simulink model "mech_pole_vault"  (Simulink 7.1)
settings: Solver=ode15s  StartTime=0.0  StopTime=5  RelTol=1e-3  AbsTol=1e-6
PreLoadFcn:
  | poleLength = 4; %m
  | poleAngle = 60;  %deg
  | poleMass = 12; %Kg
  | poleInertia = [11.9 0 0;0 11.9 0;0 0 0.0024];
  | %-----------------------------------------
  | jumperMass = 60; %Kg
  | jumperInertia = eye(3,3);
  | jumperCG = [0 -0.1 0];
  | %----------------------------------------
  | runLength = 10; %m
  | jumpHeight = 4; %m
InitFcn:
  | poleLength = 4; %m
  | poleAngle = 60;  %deg
  | poleMass = 12; %Kg
  | poleInertia = [11.9 0 0;0 11.9 0;0 0 0.0024];
  | %-----------------------------------------
  | jumperMass = 60; %Kg
  | jumperInertia = eye(3,3);
  | jumperCG = [0 -0.1 0];
  | %----------------------------------------
  | runLength = 10; %m
  | jumpHeight = 4; %m
undefined symbols (not defined in the file or in its folder): rad, s
libraries: mblibv1 x33, simulink x9
settings Model: Creator=arnav  LastModifiedBy=batserve
settings DataIOCC: OutputOption=SpecifiedOutputTimes  OutputTimes=linspace(0,5,100)  Refine=3
settings DebuggingCC: AlgebraicLoopMsg=none  SaveWithParameterizedLinksMsg=none  SignalResolutionControl=TryResolveAllWithWarning  SolverPrmCheckMsg=none  MultiTaskDSMMsg=warning  MultiTaskCondExecSysMsg=none  SigSpecEnsureSampleTimeMsg=none  ModelReferenceExtraNoncontSigs=warning  StrictBusMsg=None
settings HardwareCC: TargetBitPerLong=64  TargetEndianess=LittleEndian  TargetWordSize=64  TargetHWDeviceType=MATLAB Host  ProdEqTarget=off
settings RTWCC: SystemTargetFile=rsim.tlc  TemplateMakefile=rsim_default_tmf  Description=Rapid Simulation Target  ProcessScript=rsim_make_rtw_hook  IncludeERTFirstTime=on
settings RSimTargetCC: TargetFcnLib=ansi_tfl_tmw.mat  TargetFunctionLibrary=ANSI_C  IsPILTarget=off  EnableShiftOperators=on  PortableWordSizes=off
settings SimMechanicsCC: WarnOnRedundantConstraints=off  VisOnUpdateDiagram=on  VisDuringSimulation=on  VisConfigFile=mech_polevault.mat

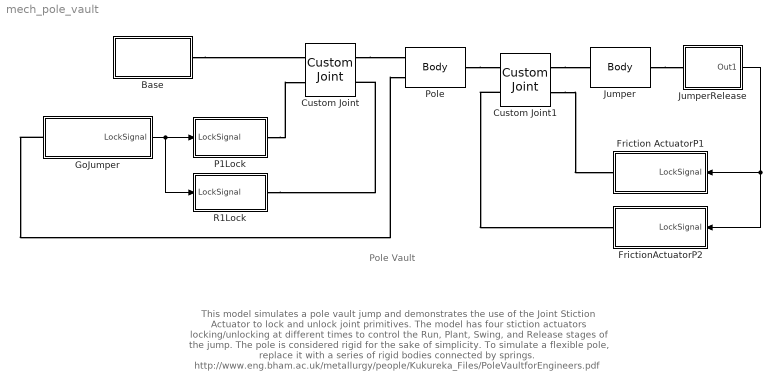
== system mech_pole_vault ==
  note: This model simulates a pole vault jump and demonstrates the use of
      | the Joint Stiction Actuator to lock and unlock joint primitives.
      | The model has four stiction actuators locking/unlocking at different times
      | to control the Run, Plant, Swing, and Release stages of the jump.
      |
      | The pole is considered rigid for the sake of simplicity.  To simulate a flexible pole,
      | replace it with a series of rigid bodies connected by springs.
      |
      | http://www.eng.bham.ac.uk/metallurgy/people/Kukureka_Files/PoleVaultforEngineers.pdf
  note: Pole Vault
  Base : Subsystem
  Custom Joint : mblibv1/Joints/Custom Joint  DialogController=MECH.DynMechDlgSource  PhysicalDomain=mechanical  SubClassName=custom_joint  LeftPortType=blob  RightPortType=blob  LConnTagsString=__newl0|SA1  RConnTagsString=__newr0|SA1  NumSAPorts=2  CutJoint=off  MarkAsCut=off  Primitives=prismatic_revolute  PrimitiveProps=P1$WORLD$[1 0 0]$prismatic#R1$WORLD$[0 0 1]$revolute  DialogClass=JointBlock  R1Axis=[0 0 1]  R2Axis=[]  R3Axis=[]  P1Axis=[1 0 0]  P2Axis=[]  P3Axis=[]  SAxis=[]
  Custom Joint1 : mblibv1/Joints/Custom Joint  DialogController=MECH.DynMechDlgSource  PhysicalDomain=mechanical  SubClassName=custom_joint  LeftPortType=blob  RightPortType=blob  LConnTagsString=__newl0|SA1  RConnTagsString=__newr0|SA1  NumSAPorts=2  CutJoint=off  MarkAsCut=off  Primitives=revolute_prismatic_prismatic  PrimitiveProps=R1$WORLD$[0 0 1]$revolute#P1$WORLD$[1 0 0]$prismatic#P2$WORLD$[0 1 0]$prismatic  DialogClass=JointBlock  R1Axis=[0 0 1]  R2Axis=[]  R3Axis=[]  P1Axis=[1 0 0]  P2Axis=[0 1 0]  P3Axis=[]  SAxis=[]
  Friction ActuatorP1 : Subsystem  Orientation=left  AncestorBlock=mech_friction/Normal Friction Actuator  mask(Normal Friction Actuator){Ckinetic=20, staticFF=20, Csforward=0.055, Csreverse=0.055, sExtActuation=on, sForces=off, primitive=P1}
      mask prompts: Ckinetic "Kinetic friction coefficient"; staticFF "Static friction coefficient"; Csforward "Forward stiction coefficient"; Csreverse "Reverse stiction coefficient"; sExtActuation "Show external actuation port"; sForces "Show kinetic and static friction ports"; primitive "Joint primitive"
      mask help:
      | Applies kinetic and static contact friction to a joint primitive. The friction force/torque is proportional to the force normal to the frictional surfaces in contact. In order for the actuated joint to be able to lock, the static friction coefficient muS must be larger than the kinetic friction coefficient muK. The friction force is mu*(normal force). The coefficient mu should be positive.
      |
      | Connect the round mechanical connection port to an actuator port on the Joint. You can friction actuate a prismatic or revolute primitive, but not a spherical primitive.
      |
      | The joint primitive menu lists all possible primitives. You must select the correct primitive after you connect the actuator to the joint.
      mask init:
      | Csforward = staticFF*Ckinetic;
      | Csreverse = staticFF*Ckinetic;
      | mech_normalFrictionActuator(gcb,'setPrimitive');
      | mech_normalFrictionActuator(gcb,'showHideActuatorSignal',sExtActuation);
      | mech_normalFrictionActuator(gcb,'showHideFrictionForces',sForces);
      settings: CopyFcn=|
      | %set_param(gcb,'LinkStatus','none');
      | %set_param(gcb,'CopyFcn','');
      mask StyleString: edit,edit,edit,edit,checkbox,checkbox,popup(P1|P2|P3|R1|R2|R3)
      mask CallbackString: ||||||%populateStictionPrimitiveList(gcb);
  FrictionActuatorP2 : Subsystem  Orientation=left  AncestorBlock=mech_friction/Normal Friction Actuator  mask(Normal Friction Actuator){Ckinetic=20, staticFF=20, Csforward=0.055, Csreverse=0.055, sExtActuation=on, sForces=off, primitive=P2}
      mask prompts: Ckinetic "Kinetic friction coefficient"; staticFF "Static friction coefficient"; Csforward "Forward stiction coefficient"; Csreverse "Reverse stiction coefficient"; sExtActuation "Show external actuation port"; sForces "Show kinetic and static friction ports"; primitive "Joint primitive"
      mask help:
      | Applies kinetic and static contact friction to a joint primitive. The friction force/torque is proportional to the force normal to the frictional surfaces in contact. In order for the actuated joint to be able to lock, the static friction coefficient muS must be larger than the kinetic friction coefficient muK. The friction force is mu*(normal force). The coefficient mu should be positive.
      |
      | Connect the round mechanical connection port to an actuator port on the Joint. You can friction actuate a prismatic or revolute primitive, but not a spherical primitive.
      |
      | The joint primitive menu lists all possible primitives. You must select the correct primitive after you connect the actuator to the joint.
      mask init: same as mech_pole_vault/Friction ActuatorP1
      settings: CopyFcn=|
      | %set_param(gcb,'LinkStatus','none');
      | %set_param(gcb,'CopyFcn','');
      mask StyleString: edit,edit,edit,edit,checkbox,checkbox,popup(P1|P2|P3|R1|R2|R3)
      mask CallbackString: ||||||%populateStictionPrimitiveList(gcb);
  GoJumper : Subsystem
  Jumper : mblibv1/Bodies/Body  DialogController=MECH.DynMechDlgSource  PhysicalDomain=mechanical  SubClassName=Unknown  LeftPortType=workingframe  RightPortType=workingframe  LConnTagsString=CS1  RConnTagsString=CG  DialogClass=MechanicalBodyBlock  Mass=jumperMass  MassUnits=kg  InertiaUnits=kg*m^2  Inertia=jumperInertia*1  Shape=Cylinder  ShapeDims=[1 1]  ShapeUnits=m  ShapeUse=false  Density=1  DensityUnits=kg/m^3  DensityUse=false  GraphicsMode=1  BodyColor=[0.5 0.5 0.5]  GraphicsObj=[]  AttachedToCS=1  CG=Right$CG$[0 -0.1 0]$CS1$CS1$m$[0 0 0]$Euler X-Y-Z$deg$WORLD$true  WorkingFrames=Left$CS1$[0 0 0]$ADJOINING$ADJOINING$m$[0 0 0]$Euler X-Y-Z$deg$WORLD$true#Right$CS2$[0 0 0]$CS1$CS1$m$[0 0 0]$Euler X-Y-Z$deg$WORLD$false  CGPos=[0 -0.1 0]  CGRot=[0 0 0]  CS0Pos=[]  CS0Rot=[]  CS1Pos=[0 0 0]  CS1Rot=[0 0 0]  CS2Pos=[0 0 0]  CS2Rot=[0 0 0]  CS3Pos=[]  CS3Rot=[]  CS4Pos=[]  CS4Rot=[]  CS5Pos=[]  CS5Rot=[]  CS6Pos=[]  CS6Rot=[]  CS7Pos=[]  CS7Rot=[]  CS8Pos=[]  CS8Rot=[]  CS9Pos=[]  CS9Rot=[]  CS10Pos=[]  CS10Rot=[]  CS11Pos=[]  CS11Rot=[]  CS12Pos=[]  CS12Rot=[]  CS13Pos=[]  CS13Rot=[]  CS14Pos=[]  CS14Rot=[]  CS15Pos=[]  CS15Rot=[]  CS16Pos=[]  CS16Rot=[]  CS17Pos=[]  CS17Rot=[]  CS18Pos=[]  CS18Rot=[]  CS19Pos=[]  CS19Rot=[]  CS20Pos=[]  CS20Rot=[]
  JumperRelease : Subsystem
  P1Lock : Subsystem
  Pole : mblibv1/Bodies/Body  DialogController=MECH.DynMechDlgSource  PhysicalDomain=mechanical  SubClassName=Unknown  LeftPortType=workingframe  RightPortType=workingframe  LConnTagsString=CS1|CS3  RConnTagsString=CS2  DialogClass=MechanicalBodyBlock  Mass=poleMass  MassUnits=kg  InertiaUnits=kg*m^2  Inertia=poleInertia  Shape=Cylinder  ShapeDims=[1 1]  ShapeUnits=m  ShapeUse=false  Density=1  DensityUnits=kg/m^3  DensityUse=false  GraphicsMode=1  BodyColor=[0.5 0.5 0.5]  GraphicsObj=[]  AttachedToCS=1  CG=Left$CG$[poleLength 0 0]/2$CS1$CS1$m$[0 90 0]$Euler X-Y-Z$deg$CS1$false  WorkingFrames=Left$CS1$[runLength 0 0]$WORLD$WORLD$m$[0 0 poleAngle]$Euler X-Y-Z$deg$WORLD$true#Left$CS3$[0 0 0]$CS1$CS1$m$[0 0 0]$Euler X-Y-Z$deg$WORLD$true#Right$CS2$[poleLength 0 0]$CS1$CS1$m$[0 0 0]$Euler X-Y-Z$deg$CS1$true  CGPos=[poleLength 0 0]/2  CGRot=[0 90 0]  CS0Pos=[]  CS0Rot=[]  CS1Pos=[runLength 0 0]  CS1Rot=[0 0 poleAngle]  CS2Pos=[poleLength 0 0]  CS2Rot=[0 0 0]  CS3Pos=[0 0 0]  CS3Rot=[0 0 0]  CS4Pos=[]  CS4Rot=[]  CS5Pos=[]  CS5Rot=[]  CS6Pos=[]  CS6Rot=[]  CS7Pos=[]  CS7Rot=[]  CS8Pos=[]  CS8Rot=[]  CS9Pos=[]  CS9Rot=[]  CS10Pos=[]  CS10Rot=[]  CS11Pos=[]  CS11Rot=[]  CS12Pos=[]  CS12Rot=[]  CS13Pos=[]  CS13Rot=[]  CS14Pos=[]  CS14Rot=[]  CS15Pos=[]  CS15Rot=[]  CS16Pos=[]  CS16Rot=[]  CS17Pos=[]  CS17Rot=[]  CS18Pos=[]  CS18Rot=[]  CS19Pos=[]  CS19Rot=[]  CS20Pos=[]  CS20Rot=[]
  R1Lock : Subsystem
  wires:
  GoJumper/1(LockSignal) -> R1Lock/1(LockSignal), P1Lock/1(LockSignal)
  JumperRelease/1(Out1) -> Friction ActuatorP1/1(LockSignal), FrictionActuatorP2/1(LockSignal)
  connections:
  Base/RConn1 -- Custom Joint/LConn1
  Custom Joint/RConn1 -- Pole/LConn1
  GoJumper/LConn1 -- Pole/LConn2
  Pole/RConn1 -- Custom Joint1/LConn1
  Custom Joint1/RConn1 -- Jumper/LConn1
  P1Lock/RConn1 -- Custom Joint/LConn2
  Jumper/RConn1 -- JumperRelease/LConn1
  R1Lock/RConn1 -- Custom Joint/RConn2
  Custom Joint1/RConn2 -- Friction ActuatorP1/RConn1
  Custom Joint1/LConn2 -- FrictionActuatorP2/RConn1

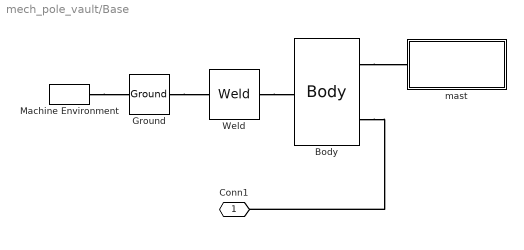
== system mech_pole_vault/Base ==
  Body : mblibv1/Bodies/Body  DialogController=MECH.DynMechDlgSource  PhysicalDomain=mechanical  SubClassName=Unknown  LeftPortType=workingframe  RightPortType=workingframe  LConnTagsString=CS1  RConnTagsString=CS4|CS2  DialogClass=MechanicalBodyBlock  Mass=30  MassUnits=kg  InertiaUnits=kg*m^2  Inertia=[1 0 0;0 0.01 0;0 0 1]*150  Shape=Cylinder  ShapeDims=[1 1]  ShapeUnits=m  ShapeUse=false  Density=1  DensityUnits=kg/m^3  DensityUse=false  GraphicsMode=1  BodyColor=[0.5 0.5 0.5]  GraphicsObj=[]  AttachedToCS=1  CG=Right$CG$[1 0 0]$CS1$CS1$m$[0 0 90]$Euler X-Y-Z$deg$WORLD$false  WorkingFrames=Right$CS4$[0 0 0]$CS1$CS1$m$[0 0 0]$Euler X-Y-Z$deg$WORLD$true#Left$CS1$[0 0 0]$ADJOINING$ADJOINING$m$[0 0 0]$Euler X-Y-Z$deg$WORLD$true#Right$CS2$[0 0 0]$CS1$CS1$m$[0 0 0]$Euler X-Y-Z$deg$WORLD$true#Right$CS3$[-3 0 0]$CS1$CS1$m$[0 0 0]$Euler X-Y-Z$deg$WORLD$false#Right$CS5$[-10 0 0]$CS1$CS1$m$[0 0 0]$Euler X-Y-Z$deg$WORLD$false#Right$CS6$[9 0 2]$CS1$CS1$m$[0 0 0]$Euler X-Y-Z$deg$WORLD$false#Right$CS7$[9 0 -2]$CS1$CS1$m$[0 0 0]$Euler X-Y-Z$deg$WORLD$false#Right$CS8$[-10 0 2]$CS1$CS1$m$[0 0 0]$Euler X-Y-Z$deg$WORLD$false#Right$CS9$[-10 0 -2]$CS1$CS1$m$[0 0 0]$Euler X-Y-Z$deg$WORLD$false  CGPos=[1 0 0]  CGRot=[0 0 90]  CS0Pos=[]  CS0Rot=[]  CS1Pos=[0 0 0]  CS1Rot=[0 0 0]  CS2Pos=[0 0 0]  CS2Rot=[0 0 0]  CS3Pos=[-3 0 0]  CS3Rot=[0 0 0]  CS4Pos=[0 0 0]  CS4Rot=[0 0 0]  CS5Pos=[-10 0 0]  CS5Rot=[0 0 0]  CS6Pos=[9 0 2]  CS6Rot=[0 0 0]  CS7Pos=[9 0 -2]  CS7Rot=[0 0 0]  CS8Pos=[-10 0 2]  CS8Rot=[0 0 0]  CS9Pos=[-10 0 -2]  CS9Rot=[0 0 0]  CS10Pos=[]  CS10Rot=[]  CS11Pos=[]  CS11Rot=[]  CS12Pos=[]  CS12Rot=[]  CS13Pos=[]  CS13Rot=[]  CS14Pos=[]  CS14Rot=[]  CS15Pos=[]  CS15Rot=[]  CS16Pos=[]  CS16Rot=[]  CS17Pos=[]  CS17Rot=[]  CS18Pos=[]  CS18Rot=[]  CS19Pos=[]  CS19Rot=[]  CS20Pos=[]  CS20Rot=[]
  Ground : mblibv1/Bodies/Ground  DialogController=MECH.DynMechDlgSource  SystemSampleTime=-1  LeftPortType=env  RightPortType=workingframe  PhysicalDomain=Mechanical  DialogClass=GroundBlock  CoordPosition=[0 0 0]  CoordPositionUnits=m  StateVectorMgrId=-1  MachineId=[0 0]  ShowEnvPort=on
  Machine Environment : mblibv1/Bodies/Machine Environment  Tag=Factory ground  DialogController=MECH.DialogSource  SystemSampleTime=-1  PortType=env  PhysicalDomain=Mechanical  DialogTemplateClass=MECH.MachineEnvironment  SyncWhenCopied=off  Gravity=[0 -9.81 0]  GravityUnits=m/s^2  GravityAsSignal=off  Dimensionality=Auto-detect  AnalysisType=Forward dynamics  LinearAssemblyTolerance=1e-3  LinearAssemblyToleranceUnits=m  AngularAssemblyTolerance=1e-3  AngularAssemblyToleranceUnits=rad  ConstraintSolverType=Stabilizing  ConstraintRelTolerance=1e-4  ConstraintAbsTolerance=1e-4  UseRobustSingularityHandling=off  RedundancyAnalysisToleranceType=Automatically select tolerance  RedundancyAnalysisTolerance=1e-14  StatePerturbationType=Fixed  PerturbationSize=1e-5  VisualizeMachine=on
  Weld : mblibv1/Joints/Weld  DialogController=MECH.DynMechDlgSource  PhysicalDomain=mechanical  SubClassName=Unknown  LeftPortType=blob  RightPortType=blob  LConnTagsString=__newl0  RConnTagsString=__newr0  NumSAPorts=0  CutJoint=off  MarkAsCut=off  Primitives=weld  PrimitiveProps=W$INERTIAL$[0 0 0]$weld  DialogClass=JointBlock  WAxis=[0 0 0]
  mast : Subsystem
  Conn1 : PMIOPort  Port=1  Side=Right
  connections:
  Weld/RConn1 -- Body/LConn1
  Machine Environment/RConn1 -- Ground/LConn1
  Ground/RConn1 -- Weld/LConn1
  Body/RConn1 -- mast/LConn1
  Body/RConn2 -- Conn1/RConn1

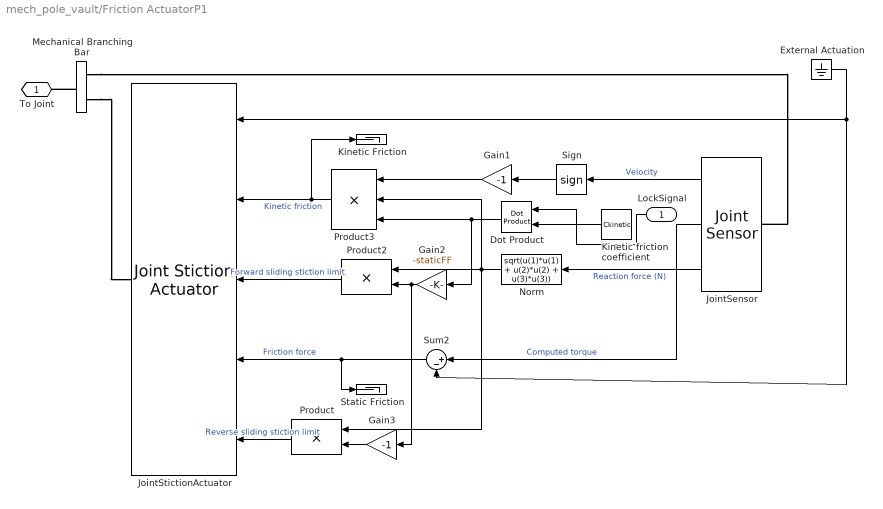
== system mech_pole_vault/Friction ActuatorP1 ==
  LockSignal : Inport  Orientation=left  OutDataType=sfix(16)  OutScaling=2^0
  Dot Product : simulink/Math Operations/Dot Product  Orientation=left  InputSameDT=on  OutDataType=sfix(16)  OutScaling=2^-10  DoSatur=off
  External Actuation : Ground
  Gain1 : Gain  Orientation=left  Gain=-1  ParameterDataType=sfix(16)  ParameterScaling=2^0  OutDataType=sfix(16)  OutScaling=2^0  SaturateOnIntegerOverflow=on  OutDataTypeStr=Inherit: Same as input  ParamDataTypeStr=Inherit: Same as input
  Gain2 : Gain  Orientation=left  Gain=-staticFF  ParameterDataType=sfix(16)  ParameterScaling=2^0  OutDataType=sfix(16)  OutScaling=2^0  SaturateOnIntegerOverflow=on  OutDataTypeStr=Inherit: Same as input  ParamDataTypeStr=Inherit: Same as input
  Gain3 : Gain  Orientation=left  Gain=-1  ParameterDataType=sfix(16)  ParameterScaling=2^0  OutDataType=sfix(16)  OutScaling=2^0  SaturateOnIntegerOverflow=on  OutDataTypeStr=Inherit: Same as input  ParamDataTypeStr=Inherit: Same as input
  JointSensor : mblibv1/Sensors &  Actuators/Joint Sensor  Orientation=left  DialogController=MECH.DynMechDlgSource  SystemSampleTime=-1  PhysicalDomain=Mechanical  PortType=blob  Muxed=off  Pose=off  Angle=off  AngleUnits=deg  ArcVelocity=on  ArcVelocityUnits=rad/s  ArcAcceleration=off  ArcAccelerationUnits=deg/s^2  CoordPosition=off  CoordPositionUnits=m  Velocity=on  VelocityUnits=m/s  Acceleration=off  AccelerationUnits=m/s^2  Quaternion=on  QuaternionDT=off  QuaternionDDT=off  QuaternionUnits=deg  OutputVector=[ 1 1 3 ]  ActiveIO=on  Width=5  DialogClass=MechanicalSensorBlock  Primitive=P1  Force=on  ForceUnits=N  Torque=on  TorqueUnits=N-m  ReferenceFrame=Absolute (INERTIAL)  ReactionSensedSide=Base  ReactionReferenceFrame=Absolute (World)  ReactionForce=on  ReactionForceUnits=N  ReactionMoment=off  ReactionMomentUnits=N-m
  JointStictionActuator : mblibv1/Sensors &  Actuators/Joint Stiction Actuator  Orientation=left  DialogController=MECH.DynMechDlgSource  SystemSampleTime=-1  PhysicalDomain=Mechanical  PortType=blob  ActuationStyle=Force  AngleUnits=deg  ArcVelocityUnits=deg/s  ArcAccelerationUnits=deg/s^2  CoordPositionUnits=m  VelocityUnits=m/s  AccelerationUnits=m/s^2  ForceUnits=N  TorqueUnits=N-m  ActiveIO=on  Width=5  DialogClass=EventActuatorBlock  Primitive=P1  FrictionalForceUnits=N  ExternalForceUnits=N  FrictionalTorqueUnits=N-m  ExternalTorqueUnits=N-m  LockingTolerance=1e-2
  Kinetic Friction : Terminator
  Kinetic friction  coefficient : Constant  Orientation=left  Value=Ckinetic  OutDataType=sfix(16)  OutScaling=2^0
  Mechanical Branching Bar : mblibv1/Utilities/Mechanical Branching Bar  DialogController=MECH.DynMechDlgSource  PhysicalDomain=mechanical  SubClassName=Unknown  LeftPortType=blob  RightPortType=blob  LConnTagsString=_newl0  RConnTagsString=SA0|SA1  DialogClass=MechanicalBranchingBarBlock  NumSAPorts=2
  Norm : Fcn  Orientation=left  Expr=sqrt(u(1)*u(1) + u(2)*u(2) + u(3)*u(3))
  Product : Product  Orientation=left  OutDataType=sfix(16)  OutScaling=2^0  SaturateOnIntegerOverflow=on  InputSameDT=on  OutDataTypeStr=Inherit: Same as first input
  Product2 : Product  Orientation=left  OutDataType=sfix(16)  OutScaling=2^0  SaturateOnIntegerOverflow=on  InputSameDT=on  OutDataTypeStr=Inherit: Same as first input
  Product3 : Product  Orientation=left  Inputs=3  OutDataType=sfix(16)  OutScaling=2^0  SaturateOnIntegerOverflow=on  InputSameDT=on  OutDataTypeStr=Inherit: Same as first input
  Sign : Signum  Orientation=left  ZeroCross=off
  Static Friction : Terminator
  Sum2 : Sum  Orientation=left  Inputs=|+-  OutDataType=sfix(16)  OutScaling=2^0  SaturateOnIntegerOverflow=on  InputSameDT=on  OutDataTypeStr=Inherit: Same as first input
  To Joint : PMIOPort  Port=1  Side=Right
  wires:
  Gain3/1 -> Product/2
  Gain2/1 -> Gain3/1, Product2/2
  LockSignal/1 -> Dot Product/1
  Dot Product/1 -> Gain2/1, Product3/3
  Kinetic friction  coefficient/1 -> Dot Product/2
  JointSensor/1 -> Sign/1  "Velocity"
  Sign/1 -> Gain1/1
  JointSensor/3 -> Norm/1  "Reaction force (N)"
  Product/1 -> JointStictionActuator/5  "Reverse sliding stiction limit"
  Product2/1 -> JointStictionActuator/3  "Forward sliding stiction limit"
  Norm/1 -> Product3/2, Product2/1, Product/1
  Gain1/1 -> Product3/1
  Product3/1 -> JointStictionActuator/2, Kinetic Friction/1  "Kinetic friction"
  JointSensor/2 -> Sum2/1  "Computed torque"
  Sum2/1 -> JointStictionActuator/4, Static Friction/1  "Friction force"
  External Actuation/1 -> JointStictionActuator/1, Sum2/2
  connections:
  Mechanical Branching Bar/RConn2 -- JointStictionActuator/RConn1
  Mechanical Branching Bar/LConn1 -- To Joint/RConn1
  Mechanical Branching Bar/RConn1 -- JointSensor/LConn1

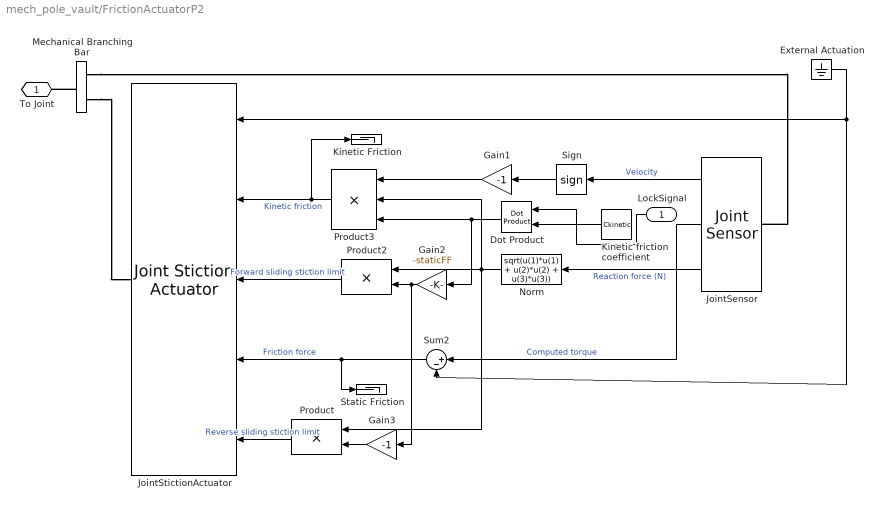
== system mech_pole_vault/FrictionActuatorP2 ==
  LockSignal : Inport  Orientation=left  OutDataType=sfix(16)  OutScaling=2^0
  Dot Product : simulink/Math Operations/Dot Product  Orientation=left  InputSameDT=on  OutDataType=sfix(16)  OutScaling=2^-10  DoSatur=off
  External Actuation : Ground
  Gain1 : Gain  Orientation=left  Gain=-1  ParameterDataType=sfix(16)  ParameterScaling=2^0  OutDataType=sfix(16)  OutScaling=2^0  SaturateOnIntegerOverflow=on  OutDataTypeStr=Inherit: Same as input  ParamDataTypeStr=Inherit: Same as input
  Gain2 : Gain  Orientation=left  Gain=-staticFF  ParameterDataType=sfix(16)  ParameterScaling=2^0  OutDataType=sfix(16)  OutScaling=2^0  SaturateOnIntegerOverflow=on  OutDataTypeStr=Inherit: Same as input  ParamDataTypeStr=Inherit: Same as input
  Gain3 : Gain  Orientation=left  Gain=-1  ParameterDataType=sfix(16)  ParameterScaling=2^0  OutDataType=sfix(16)  OutScaling=2^0  SaturateOnIntegerOverflow=on  OutDataTypeStr=Inherit: Same as input  ParamDataTypeStr=Inherit: Same as input
  JointSensor : mblibv1/Sensors &  Actuators/Joint Sensor  Orientation=left  DialogController=MECH.DynMechDlgSource  SystemSampleTime=-1  PhysicalDomain=Mechanical  PortType=blob  Muxed=off  Pose=off  Angle=off  AngleUnits=deg  ArcVelocity=on  ArcVelocityUnits=rad/s  ArcAcceleration=off  ArcAccelerationUnits=deg/s^2  CoordPosition=off  CoordPositionUnits=m  Velocity=on  VelocityUnits=m/s  Acceleration=off  AccelerationUnits=m/s^2  Quaternion=on  QuaternionDT=off  QuaternionDDT=off  QuaternionUnits=deg  OutputVector=[ 1 1 3 ]  ActiveIO=on  Width=5  DialogClass=MechanicalSensorBlock  Primitive=P2  Force=on  ForceUnits=N  Torque=on  TorqueUnits=N-m  ReferenceFrame=Absolute (INERTIAL)  ReactionSensedSide=Base  ReactionReferenceFrame=Absolute (World)  ReactionForce=on  ReactionForceUnits=N  ReactionMoment=off  ReactionMomentUnits=N-m
  JointStictionActuator : mblibv1/Sensors &  Actuators/Joint Stiction Actuator  Orientation=left  DialogController=MECH.DynMechDlgSource  SystemSampleTime=-1  PhysicalDomain=Mechanical  PortType=blob  ActuationStyle=Force  AngleUnits=deg  ArcVelocityUnits=deg/s  ArcAccelerationUnits=deg/s^2  CoordPositionUnits=m  VelocityUnits=m/s  AccelerationUnits=m/s^2  ForceUnits=N  TorqueUnits=N-m  ActiveIO=on  Width=5  DialogClass=EventActuatorBlock  Primitive=P2  FrictionalForceUnits=N  ExternalForceUnits=N  FrictionalTorqueUnits=N-m  ExternalTorqueUnits=N-m  LockingTolerance=1e-2
  Kinetic Friction : Terminator
  Kinetic friction  coefficient : Constant  Orientation=left  Value=Ckinetic  OutDataType=sfix(16)  OutScaling=2^0
  Mechanical Branching Bar : mblibv1/Utilities/Mechanical Branching Bar  DialogController=MECH.DynMechDlgSource  PhysicalDomain=mechanical  SubClassName=Unknown  LeftPortType=blob  RightPortType=blob  LConnTagsString=_newl0  RConnTagsString=SA0|SA1  DialogClass=MechanicalBranchingBarBlock  NumSAPorts=2
  Norm : Fcn  Orientation=left  Expr=sqrt(u(1)*u(1) + u(2)*u(2) + u(3)*u(3))
  Product : Product  Orientation=left  OutDataType=sfix(16)  OutScaling=2^0  SaturateOnIntegerOverflow=on  InputSameDT=on  OutDataTypeStr=Inherit: Same as first input
  Product2 : Product  Orientation=left  OutDataType=sfix(16)  OutScaling=2^0  SaturateOnIntegerOverflow=on  InputSameDT=on  OutDataTypeStr=Inherit: Same as first input
  Product3 : Product  Orientation=left  Inputs=3  OutDataType=sfix(16)  OutScaling=2^0  SaturateOnIntegerOverflow=on  InputSameDT=on  OutDataTypeStr=Inherit: Same as first input
  Sign : Signum  Orientation=left  ZeroCross=off
  Static Friction : Terminator
  Sum2 : Sum  Orientation=left  Inputs=|+-  OutDataType=sfix(16)  OutScaling=2^0  SaturateOnIntegerOverflow=on  InputSameDT=on  OutDataTypeStr=Inherit: Same as first input
  To Joint : PMIOPort  Port=1  Side=Right
  wires:
  External Actuation/1 -> Sum2/2, JointStictionActuator/1
  Sum2/1 -> Static Friction/1, JointStictionActuator/4  "Friction force"
  JointSensor/2 -> Sum2/1  "Computed torque"
  Product3/1 -> Kinetic Friction/1, JointStictionActuator/2  "Kinetic friction"
  Gain1/1 -> Product3/1
  Norm/1 -> Product/1, Product2/1, Product3/2
  Product2/1 -> JointStictionActuator/3  "Forward sliding stiction limit"
  Product/1 -> JointStictionActuator/5  "Reverse sliding stiction limit"
  JointSensor/3 -> Norm/1  "Reaction force (N)"
  Sign/1 -> Gain1/1
  JointSensor/1 -> Sign/1  "Velocity"
  Kinetic friction  coefficient/1 -> Dot Product/2
  Dot Product/1 -> Product3/3, Gain2/1
  LockSignal/1 -> Dot Product/1
  Gain2/1 -> Product2/2, Gain3/1
  Gain3/1 -> Product/2
  connections:
  Mechanical Branching Bar/RConn1 -- JointSensor/LConn1
  Mechanical Branching Bar/LConn1 -- To Joint/RConn1
  Mechanical Branching Bar/RConn2 -- JointStictionActuator/RConn1

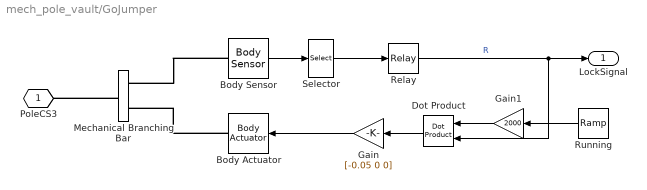
== system mech_pole_vault/GoJumper ==
  Body Actuator : mblibv1/Sensors &  Actuators/Body Actuator  Orientation=left  DialogController=MECH.DynMechDlgSource  SystemSampleTime=-1  PhysicalDomain=Mechanical  PortType=blob  ActuationStyle=Force  AngleUnits=deg  ArcVelocityUnits=deg/s  ArcAccelerationUnits=deg/s^2  CoordPositionUnits=m  VelocityUnits=m/s  AccelerationUnits=m/s^2  ForceUnits=N  TorqueUnits=N-m  ActiveIO=on  Width=3  DialogClass=MechanicalActuatorBlock  ReferenceFrame=Absolute (World)  Angle=off  CoordPosition=on  Force=on  Torque=off
  Body Sensor : mblibv1/Sensors &  Actuators/Body Sensor  DialogController=MECH.DynMechDlgSource  SystemSampleTime=-1  PhysicalDomain=Mechanical  PortType=blob  Muxed=off  Pose=off  Angle=on  AngleUnits=deg  ArcVelocity=off  ArcVelocityUnits=deg/s  ArcAcceleration=off  ArcAccelerationUnits=deg/s^2  CoordPosition=on  CoordPositionUnits=m  Velocity=off  VelocityUnits=m/s  Acceleration=off  AccelerationUnits=m/s^2  Quaternion=on  QuaternionDT=off  QuaternionDDT=off  QuaternionUnits=off  OutputVector=[ 3 ]  ActiveIO=on  Width=3  DialogClass=MechanicalSensorBlock  ReferenceFrame=Absolute (World)
  Dot Product : simulink/Math Operations/Dot Product  Orientation=left  InputSameDT=on  OutDataType=sfix(16)  OutScaling=2^-10  DoSatur=off
  Gain : Gain  Orientation=left  Gain=[-0.05 0 0]  ParameterDataType=sfix(16)  ParameterScaling=2^0  OutDataType=sfix(16)  OutScaling=2^0
  Gain1 : Gain  Orientation=left  Gain=2000  ParameterDataType=sfix(16)  ParameterScaling=2^0  OutDataType=sfix(16)  OutScaling=2^0
  Mechanical Branching Bar : mblibv1/Utilities/Mechanical Branching Bar  DialogController=MECH.DynMechDlgSource  PhysicalDomain=mechanical  SubClassName=Unknown  LeftPortType=blob  RightPortType=blob  LConnTagsString=_newl0  RConnTagsString=SA0|SA1  DialogClass=MechanicalBranchingBarBlock  NumSAPorts=2
  Relay : Relay  OnSwitchValue=runLength  OffSwitchValue=0  OutDataType=sfix(16)  OutScaling=2^0
  Running : simulink/Sources/Ramp  Orientation=left  SystemSampleTime=-1  slope=2  start=0  X0=1
  Selector : Selector  InputPortWidth=3  IndexOptions=Index vector (dialog)  Indices=[1]  OutputSizes=1
  PoleCS3 : PMIOPort  Tag=PMCPort  Port=1  Side=Left
  LockSignal : Outport  OutDataType=sfix(16)  OutScaling=2^0  InitialOutput=0
  wires:
  Selector/1 -> Relay/1
  Body Sensor/1 -> Selector/1
  Gain/1 -> Body Actuator/1
  Dot Product/1 -> Gain/1
  Running/1 -> Gain1/1
  Relay/1 -> LockSignal/1, Dot Product/2  "R"
  Gain1/1 -> Dot Product/1
  connections:
  Mechanical Branching Bar/LConn1 -- PoleCS3/RConn1
  Body Actuator/RConn1 -- Mechanical Branching Bar/RConn2
  Body Sensor/LConn1 -- Mechanical Branching Bar/RConn1

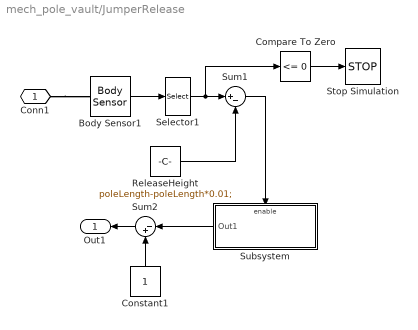
== system mech_pole_vault/JumperRelease ==
  Body Sensor1 : mblibv1/Sensors &  Actuators/Body Sensor  DialogController=MECH.DynMechDlgSource  SystemSampleTime=-1  PhysicalDomain=Mechanical  PortType=blob  Muxed=off  Pose=off  Angle=on  AngleUnits=deg  ArcVelocity=off  ArcVelocityUnits=deg/s  ArcAcceleration=off  ArcAccelerationUnits=deg/s^2  CoordPosition=on  CoordPositionUnits=m  Velocity=off  VelocityUnits=m/s  Acceleration=off  AccelerationUnits=m/s^2  Quaternion=on  QuaternionDT=off  QuaternionDDT=off  QuaternionUnits=off  OutputVector=[ 3 ]  ActiveIO=on  Width=3  DialogClass=MechanicalSensorBlock  ReferenceFrame=Absolute (World)
  Compare To Zero : simulink/Logic and Bit Operations/Compare To Zero  SystemSampleTime=-1  relop=<=  LogicOutDataTypeMode=boolean
  Constant1 : Constant  Orientation=up  OutDataType=sfix(16)  OutScaling=2^0
  ReleaseHeight : Constant  Value=poleLength-poleLength*0.01;  OutDataType=sfix(16)  OutScaling=2^0
  Selector1 : Selector  InputPortWidth=3  IndexOptions=Index vector (dialog)  Indices=[2]  OutputSizes=1
  Stop Simulation : Stop
  Subsystem : Subsystem  Orientation=left  TreatAsAtomicUnit=on
  Sum1 : Sum  Inputs=|+-  OutDataType=sfix(16)  OutScaling=2^0  SaturateOnIntegerOverflow=on
  Sum2 : Sum  Orientation=left  Inputs=|-+  OutDataType=sfix(16)  OutScaling=2^0  SaturateOnIntegerOverflow=on
  Conn1 : PMIOPort  Port=1  Side=Left
  Out1 : Outport  Orientation=left  OutDataType=sfix(16)  OutScaling=2^0
  wires:
  Body Sensor1/1 -> Selector1/1
  Selector1/1 -> Sum1/1, Compare To Zero/1
  ReleaseHeight/1 -> Sum1/2
  Sum1/1 -> Subsystem/Enable
  Subsystem/1(Out1) -> Sum2/1
  Constant1/1 -> Sum2/2
  Sum2/1 -> Out1/1
  Compare To Zero/1 -> Stop Simulation/1
  connections:
  Conn1/RConn1 -- Body Sensor1/LConn1

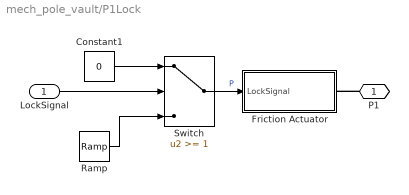
== system mech_pole_vault/P1Lock ==
  LockSignal : Inport  OutDataType=sfix(16)  OutScaling=2^0
  Constant1 : Constant  Value=0  OutDataType=sfix(16)  OutScaling=2^0
  Friction Actuator : Subsystem  AncestorBlock=mech_friction/Normal Friction Actuator  mask(Normal Friction Actuator){Ckinetic=1, staticFF=5, Csforward=0.055, Csreverse=0.055, sExtActuation=on, sForces=off, primitive=P1}
      mask prompts: Ckinetic "Kinetic friction coefficient"; staticFF "Static friction coefficient"; Csforward "Forward stiction coefficient"; Csreverse "Reverse stiction coefficient"; sExtActuation "Show external actuation port"; sForces "Show kinetic and static friction ports"; primitive "Joint primitive"
      mask help:
      | Applies kinetic and static contact friction to a joint primitive. The friction force/torque is proportional to the force normal to the frictional surfaces in contact. In order for the actuated joint to be able to lock, the static friction coefficient muS must be larger than the kinetic friction coefficient muK. The friction force is mu*(normal force). The coefficient mu should be positive.
      |
      | Connect the round mechanical connection port to an actuator port on the Joint. You can friction actuate a prismatic or revolute primitive, but not a spherical primitive.
      |
      | The joint primitive menu lists all possible primitives. You must select the correct primitive after you connect the actuator to the joint.
      mask init: same as mech_pole_vault/Friction ActuatorP1
      settings: CopyFcn=|
      | %set_param(gcb,'LinkStatus','none');
      | %set_param(gcb,'CopyFcn','');
      mask StyleString: edit,edit,edit,edit,checkbox,checkbox,popup(P1|P2|P3|R1|R2|R3)
      mask CallbackString: ||||||%populateStictionPrimitiveList(gcb);
  Ramp : simulink/Sources/Ramp  SystemSampleTime=-1  slope=1  start=2  X0=0
  Switch : Switch  Threshold=1
  P1 : PMIOPort  Orientation=left  Port=1  Side=Right
  wires:
  Constant1/1 -> Switch/1
  Ramp/1 -> Switch/3
  Switch/1 -> Friction Actuator/1(LockSignal)  "P"
  LockSignal/1 -> Switch/2
  connections:
  P1/RConn1 -- Friction Actuator/RConn1

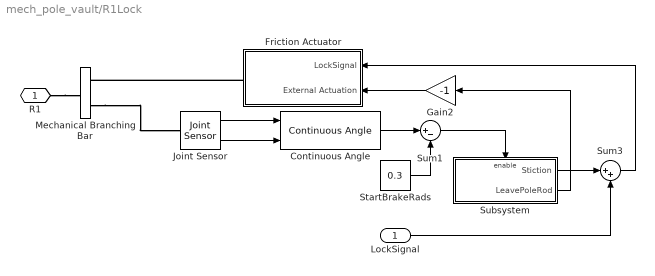
== system mech_pole_vault/R1Lock ==
  LockSignal : Inport  OutDataType=sfix(16)  OutScaling=2^0
  Continuous Angle : mblibv1/Utilities/Continuous Angle  Tag=Factory continuousAngle  SystemSampleTime=-1  rad=rad  rads=rad/s
  Friction Actuator : Subsystem  Orientation=left  AncestorBlock=mech_friction/Normal Friction Actuator  mask(Normal Friction Actuator){Ckinetic=1.2, staticFF=5, Csforward=0.055, Csreverse=0.055, sExtActuation=on, sForces=off, primitive=R1}
      mask prompts: Ckinetic "Kinetic friction coefficient"; staticFF "Static friction coefficient"; Csforward "Forward stiction coefficient"; Csreverse "Reverse stiction coefficient"; sExtActuation "Show external actuation port"; sForces "Show kinetic and static friction ports"; primitive "Joint primitive"
      mask help:
      | Applies kinetic and static contact friction to a joint primitive. The friction force/torque is proportional to the force normal to the frictional surfaces in contact. In order for the actuated joint to be able to lock, the static friction coefficient muS must be larger than the kinetic friction coefficient muK. The friction force is mu*(normal force). The coefficient mu should be positive.
      |
      | Connect the round mechanical connection port to an actuator port on the Joint. You can friction actuate a prismatic or revolute primitive, but not a spherical primitive.
      |
      | The joint primitive menu lists all possible primitives. You must select the correct primitive after you connect the actuator to the joint.
      mask init: same as mech_pole_vault/Friction ActuatorP1
      settings: CopyFcn=|
      | %set_param(gcb,'LinkStatus','none');
      | %set_param(gcb,'CopyFcn','');
      mask StyleString: edit,edit,edit,edit,checkbox,checkbox,popup(P1|P2|P3|R1|R2|R3)
      mask CallbackString: ||||||%populateStictionPrimitiveList(gcb);
  Gain2 : Gain  Orientation=left  Gain=-1  ParameterDataType=sfix(16)  ParameterScaling=2^0  OutDataType=sfix(16)  OutScaling=2^0  SaturateOnIntegerOverflow=on  OutDataTypeStr=Inherit: Same as input  ParamDataTypeStr=Inherit: Same as input
  Joint Sensor : mblibv1/Sensors &  Actuators/Joint Sensor  DialogController=MECH.DynMechDlgSource  SystemSampleTime=-1  PhysicalDomain=Mechanical  PortType=blob  Muxed=off  Pose=off  Angle=on  AngleUnits=rad  ArcVelocity=on  ArcVelocityUnits=rad/s  ArcAcceleration=off  ArcAccelerationUnits=deg/s^2  CoordPosition=on  CoordPositionUnits=m  Velocity=on  VelocityUnits=m/s  Acceleration=off  AccelerationUnits=m/s^2  Quaternion=on  QuaternionDT=off  QuaternionDDT=off  QuaternionUnits=off  OutputVector=[ 1 1 ]  ActiveIO=on  Width=2  DialogClass=MechanicalSensorBlock  Primitive=R1  Force=off  ForceUnits=N  Torque=off  TorqueUnits=N-m  ReferenceFrame=Absolute (INERTIAL)  ReactionSensedSide=Base  ReactionReferenceFrame=Absolute (World)  ReactionForce=off  ReactionForceUnits=N  ReactionMoment=off  ReactionMomentUnits=N-m
  Mechanical Branching Bar : mblibv1/Utilities/Mechanical Branching Bar  DialogController=MECH.DynMechDlgSource  PhysicalDomain=mechanical  SubClassName=Unknown  LeftPortType=blob  RightPortType=blob  LConnTagsString=_newl0  RConnTagsString=SA0|SA1  DialogClass=MechanicalBranchingBarBlock  NumSAPorts=2
  StartBrakeRads : Constant  Value=0.3  OutDataType=sfix(16)  OutScaling=2^0
  Subsystem : Subsystem  TreatAsAtomicUnit=on
  Sum1 : Sum  Inputs=|+-  OutDataType=sfix(16)  OutScaling=2^0  SaturateOnIntegerOverflow=on
  Sum3 : Sum  Inputs=|++  OutDataType=sfix(16)  OutScaling=2^0  SaturateOnIntegerOverflow=on
  R1 : PMIOPort  Port=1  Side=Right
  wires:
  Joint Sensor/1 -> Continuous Angle/1
  Joint Sensor/2 -> Continuous Angle/2
  StartBrakeRads/1 -> Sum1/2
  Sum1/1 -> Subsystem/Enable
  Continuous Angle/1 -> Sum1/1
  Subsystem/1(Stiction) -> Sum3/1
  LockSignal/1 -> Sum3/2
  Gain2/1 -> Friction Actuator/2(External Actuation)
  Subsystem/2(LeavePoleRod) -> Gain2/1
  Sum3/1 -> Friction Actuator/1(LockSignal)
  connections:
  Mechanical Branching Bar/RConn2 -- Joint Sensor/LConn1
  R1/RConn1 -- Mechanical Branching Bar/LConn1
  Friction Actuator/RConn1 -- Mechanical Branching Bar/RConn1

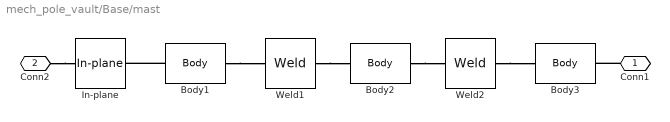
== system mech_pole_vault/Base/mast ==
  Body1 : mblibv1/Bodies/Body  DialogController=MECH.DynMechDlgSource  PhysicalDomain=mechanical  SubClassName=Unknown  LeftPortType=workingframe  RightPortType=workingframe  LConnTagsString=CS1  RConnTagsString=CS2  DialogClass=MechanicalBodyBlock  Mass=10  MassUnits=kg  InertiaUnits=kg*m^2  Inertia=[1 0 0;0 0.01 0;0 0 1]*10  Shape=Cylinder  ShapeDims=[1 1]  ShapeUnits=m  ShapeUse=false  Density=1  DensityUnits=kg/m^3  DensityUse=false  GraphicsMode=1  BodyColor=[0.5 0.5 0.5]  GraphicsObj=[]  AttachedToCS=1  CG=Left$CG$[0 jumpHeight 0]/2$CS1$CS1$m$[0 0 0]$Euler X-Y-Z$deg$WORLD$false  WorkingFrames=Left$CS1$[-3.5 0 2]$ADJOINING$ADJOINING$m$[0 0 0]$Euler X-Y-Z$deg$WORLD$true#Right$CS2$[0 jumpHeight 0]$CS1$CS1$m$[0 0 0]$Euler X-Y-Z$deg$WORLD$true  CGPos=[0 jumpHeight 0]/2  CGRot=[0 0 0]  CS0Pos=[]  CS0Rot=[]  CS1Pos=[-3.5 0 2]  CS1Rot=[0 0 0]  CS2Pos=[0 jumpHeight 0]  CS2Rot=[0 0 0]  CS3Pos=[]  CS3Rot=[]  CS4Pos=[]  CS4Rot=[]  CS5Pos=[]  CS5Rot=[]  CS6Pos=[]  CS6Rot=[]  CS7Pos=[]  CS7Rot=[]  CS8Pos=[]  CS8Rot=[]  CS9Pos=[]  CS9Rot=[]  CS10Pos=[]  CS10Rot=[]  CS11Pos=[]  CS11Rot=[]  CS12Pos=[]  CS12Rot=[]  CS13Pos=[]  CS13Rot=[]  CS14Pos=[]  CS14Rot=[]  CS15Pos=[]  CS15Rot=[]  CS16Pos=[]  CS16Rot=[]  CS17Pos=[]  CS17Rot=[]  CS18Pos=[]  CS18Rot=[]  CS19Pos=[]  CS19Rot=[]  CS20Pos=[]  CS20Rot=[]
  Body2 : mblibv1/Bodies/Body  DialogController=MECH.DynMechDlgSource  PhysicalDomain=mechanical  SubClassName=Unknown  LeftPortType=workingframe  RightPortType=workingframe  LConnTagsString=CS1  RConnTagsString=CS2  DialogClass=MechanicalBodyBlock  Mass=10  MassUnits=kg  InertiaUnits=kg*m^2  Inertia=[1 0 0;0 0.01 0;0 0 1]*10  Shape=Cylinder  ShapeDims=[1 1]  ShapeUnits=m  ShapeUse=false  Density=1  DensityUnits=kg/m^3  DensityUse=false  GraphicsMode=1  BodyColor=[0.5 0.5 0.5]  GraphicsObj=[]  AttachedToCS=1  CG=Left$CG$[0 0 -2]$CS1$CS1$m$[90 0 0]$Euler X-Y-Z$deg$WORLD$false  WorkingFrames=Left$CS1$[0 0 0]$ADJOINING$ADJOINING$m$[0 0 0]$Euler X-Y-Z$deg$WORLD$true#Right$CS2$[0 0 -4]$CS1$CS1$m$[0 0 0]$Euler X-Y-Z$deg$WORLD$true  CGPos=[0 0 -2]  CGRot=[90 0 0]  CS0Pos=[]  CS0Rot=[]  CS1Pos=[0 0 0]  CS1Rot=[0 0 0]  CS2Pos=[0 0 -4]  CS2Rot=[0 0 0]  CS3Pos=[]  CS3Rot=[]  CS4Pos=[]  CS4Rot=[]  CS5Pos=[]  CS5Rot=[]  CS6Pos=[]  CS6Rot=[]  CS7Pos=[]  CS7Rot=[]  CS8Pos=[]  CS8Rot=[]  CS9Pos=[]  CS9Rot=[]  CS10Pos=[]  CS10Rot=[]  CS11Pos=[]  CS11Rot=[]  CS12Pos=[]  CS12Rot=[]  CS13Pos=[]  CS13Rot=[]  CS14Pos=[]  CS14Rot=[]  CS15Pos=[]  CS15Rot=[]  CS16Pos=[]  CS16Rot=[]  CS17Pos=[]  CS17Rot=[]  CS18Pos=[]  CS18Rot=[]  CS19Pos=[]  CS19Rot=[]  CS20Pos=[]  CS20Rot=[]
  Body3 : mblibv1/Bodies/Body  DialogController=MECH.DynMechDlgSource  PhysicalDomain=mechanical  SubClassName=Unknown  LeftPortType=workingframe  RightPortType=workingframe  LConnTagsString=CS1  RConnTagsString=CS2  DialogClass=MechanicalBodyBlock  Mass=10  MassUnits=kg  InertiaUnits=kg*m^2  Inertia=[1 0 0;0 0.01 0;0 0 1]*10  Shape=Cylinder  ShapeDims=[1 1]  ShapeUnits=m  ShapeUse=false  Density=1  DensityUnits=kg/m^3  DensityUse=false  GraphicsMode=1  BodyColor=[0.5 0.5 0.5]  GraphicsObj=[]  AttachedToCS=1  CG=Left$CG$[0 -jumpHeight 0]/2$CS1$CS1$m$[0 0 0]$Euler X-Y-Z$deg$WORLD$false  WorkingFrames=Left$CS1$[0 0 0]$ADJOINING$ADJOINING$m$[0 0 0]$Euler X-Y-Z$deg$WORLD$true#Right$CS2$[0 -jumpHeight 0]$CS1$CS1$m$[0 0 0]$Euler X-Y-Z$deg$WORLD$true  CGPos=[0 -jumpHeight 0]/2  CGRot=[0 0 0]  CS0Pos=[]  CS0Rot=[]  CS1Pos=[0 0 0]  CS1Rot=[0 0 0]  CS2Pos=[0 -jumpHeight 0]  CS2Rot=[0 0 0]  CS3Pos=[]  CS3Rot=[]  CS4Pos=[]  CS4Rot=[]  CS5Pos=[]  CS5Rot=[]  CS6Pos=[]  CS6Rot=[]  CS7Pos=[]  CS7Rot=[]  CS8Pos=[]  CS8Rot=[]  CS9Pos=[]  CS9Rot=[]  CS10Pos=[]  CS10Rot=[]  CS11Pos=[]  CS11Rot=[]  CS12Pos=[]  CS12Rot=[]  CS13Pos=[]  CS13Rot=[]  CS14Pos=[]  CS14Rot=[]  CS15Pos=[]  CS15Rot=[]  CS16Pos=[]  CS16Rot=[]  CS17Pos=[]  CS17Rot=[]  CS18Pos=[]  CS18Rot=[]  CS19Pos=[]  CS19Rot=[]  CS20Pos=[]  CS20Rot=[]
  In-plane : mblibv1/Joints/In-plane  DialogController=MECH.DynMechDlgSource  PhysicalDomain=mechanical  SubClassName=Unknown  LeftPortType=blob  RightPortType=blob  LConnTagsString=__newl0  RConnTagsString=__newr0  NumSAPorts=0  CutJoint=off  MarkAsCut=off  Primitives=prismatic_prismatic  PrimitiveProps=P1$WORLD$[1 0 0]$prismatic#P2$WORLD$[0 0 1]$prismatic  DialogClass=JointBlock  P1Axis=[1 0 0]  P2Axis=[0 0 1]
  Weld1 : mblibv1/Joints/Weld  DialogController=MECH.DynMechDlgSource  PhysicalDomain=mechanical  SubClassName=Unknown  LeftPortType=blob  RightPortType=blob  LConnTagsString=__newl0  RConnTagsString=__newr0  NumSAPorts=0  CutJoint=off  MarkAsCut=off  Primitives=weld  PrimitiveProps=W$INERTIAL$[0 0 0]$weld  DialogClass=JointBlock  WAxis=[0 0 0]
  Weld2 : mblibv1/Joints/Weld  DialogController=MECH.DynMechDlgSource  PhysicalDomain=mechanical  SubClassName=Unknown  LeftPortType=blob  RightPortType=blob  LConnTagsString=__newl0  RConnTagsString=__newr0  NumSAPorts=0  CutJoint=off  MarkAsCut=off  Primitives=weld  PrimitiveProps=W$INERTIAL$[0 0 0]$weld  DialogClass=JointBlock  WAxis=[0 0 0]
  Conn1 : PMIOPort  Orientation=left  Port=1  Side=Right
  Conn2 : PMIOPort  Port=2  Side=Left
  connections:
  Body1/LConn1 -- In-plane/RConn1
  Body1/RConn1 -- Weld1/LConn1
  Weld1/RConn1 -- Body2/LConn1
  Body2/RConn1 -- Weld2/LConn1
  Weld2/RConn1 -- Body3/LConn1
  Conn1/RConn1 -- Body3/RConn1
  Conn2/RConn1 -- In-plane/LConn1

== system mech_pole_vault/JumperRelease/Subsystem ==
  Enable : EnablePort
  Constant4 : Constant  OutDataType=sfix(16)  OutScaling=2^0
  Out1 : Outport  OutDataType=sfix(16)  OutScaling=2^0  InitialOutput=0
  wires:
  Constant4/1 -> Out1/1

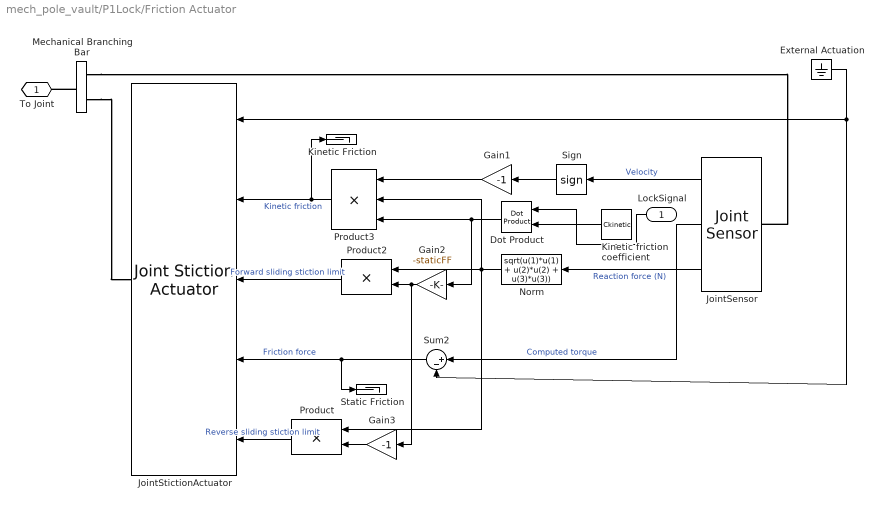
== system mech_pole_vault/P1Lock/Friction Actuator ==
  LockSignal : Inport  Orientation=left  OutDataType=sfix(16)  OutScaling=2^0
  Dot Product : simulink/Math Operations/Dot Product  Orientation=left  InputSameDT=on  OutDataType=sfix(16)  OutScaling=2^-10  DoSatur=off
  External Actuation : Ground
  Gain1 : Gain  Orientation=left  Gain=-1  ParameterDataType=sfix(16)  ParameterScaling=2^0  OutDataType=sfix(16)  OutScaling=2^0  SaturateOnIntegerOverflow=on  OutDataTypeStr=Inherit: Same as input  ParamDataTypeStr=Inherit: Same as input
  Gain2 : Gain  Orientation=left  Gain=-staticFF  ParameterDataType=sfix(16)  ParameterScaling=2^0  OutDataType=sfix(16)  OutScaling=2^0  SaturateOnIntegerOverflow=on  OutDataTypeStr=Inherit: Same as input  ParamDataTypeStr=Inherit: Same as input
  Gain3 : Gain  Orientation=left  Gain=-1  ParameterDataType=sfix(16)  ParameterScaling=2^0  OutDataType=sfix(16)  OutScaling=2^0  SaturateOnIntegerOverflow=on  OutDataTypeStr=Inherit: Same as input  ParamDataTypeStr=Inherit: Same as input
  JointSensor : mblibv1/Sensors &  Actuators/Joint Sensor  Orientation=left  DialogController=MECH.DynMechDlgSource  SystemSampleTime=-1  PhysicalDomain=Mechanical  PortType=blob  Muxed=off  Pose=off  Angle=off  AngleUnits=deg  ArcVelocity=on  ArcVelocityUnits=rad/s  ArcAcceleration=off  ArcAccelerationUnits=deg/s^2  CoordPosition=off  CoordPositionUnits=m  Velocity=on  VelocityUnits=m/s  Acceleration=off  AccelerationUnits=m/s^2  Quaternion=on  QuaternionDT=off  QuaternionDDT=off  QuaternionUnits=deg  OutputVector=[ 1 1 3 ]  ActiveIO=on  Width=5  DialogClass=MechanicalSensorBlock  Primitive=P1  Force=on  ForceUnits=N  Torque=on  TorqueUnits=N-m  ReferenceFrame=Absolute (INERTIAL)  ReactionSensedSide=Base  ReactionReferenceFrame=Absolute (World)  ReactionForce=on  ReactionForceUnits=N  ReactionMoment=off  ReactionMomentUnits=N-m
  JointStictionActuator : mblibv1/Sensors &  Actuators/Joint Stiction Actuator  Orientation=left  DialogController=MECH.DynMechDlgSource  SystemSampleTime=-1  PhysicalDomain=Mechanical  PortType=blob  ActuationStyle=Force  AngleUnits=deg  ArcVelocityUnits=deg/s  ArcAccelerationUnits=deg/s^2  CoordPositionUnits=m  VelocityUnits=m/s  AccelerationUnits=m/s^2  ForceUnits=N  TorqueUnits=N-m  ActiveIO=on  Width=5  DialogClass=EventActuatorBlock  Primitive=P1  FrictionalForceUnits=N  ExternalForceUnits=N  FrictionalTorqueUnits=N-m  ExternalTorqueUnits=N-m  LockingTolerance=1e-2
  Kinetic Friction : Terminator
  Kinetic friction  coefficient : Constant  Orientation=left  Value=Ckinetic  OutDataType=sfix(16)  OutScaling=2^0
  Mechanical Branching Bar : mblibv1/Utilities/Mechanical Branching Bar  DialogController=MECH.DynMechDlgSource  PhysicalDomain=mechanical  SubClassName=Unknown  LeftPortType=blob  RightPortType=blob  LConnTagsString=_newl0  RConnTagsString=SA0|SA1  DialogClass=MechanicalBranchingBarBlock  NumSAPorts=2
  Norm : Fcn  Orientation=left  Expr=sqrt(u(1)*u(1) + u(2)*u(2) + u(3)*u(3))
  Product : Product  Orientation=left  OutDataType=sfix(16)  OutScaling=2^0  SaturateOnIntegerOverflow=on  InputSameDT=on  OutDataTypeStr=Inherit: Same as first input
  Product2 : Product  Orientation=left  OutDataType=sfix(16)  OutScaling=2^0  SaturateOnIntegerOverflow=on  InputSameDT=on  OutDataTypeStr=Inherit: Same as first input
  Product3 : Product  Orientation=left  Inputs=3  OutDataType=sfix(16)  OutScaling=2^0  SaturateOnIntegerOverflow=on  InputSameDT=on  OutDataTypeStr=Inherit: Same as first input
  Sign : Signum  Orientation=left  ZeroCross=off
  Static Friction : Terminator
  Sum2 : Sum  Orientation=left  Inputs=|+-  OutDataType=sfix(16)  OutScaling=2^0  SaturateOnIntegerOverflow=on  InputSameDT=on  OutDataTypeStr=Inherit: Same as first input
  To Joint : PMIOPort  Port=1  Side=Right
  wires:
  Gain3/1 -> Product/2
  Gain2/1 -> Gain3/1, Product2/2
  LockSignal/1 -> Dot Product/1
  Dot Product/1 -> Gain2/1, Product3/3
  Kinetic friction  coefficient/1 -> Dot Product/2
  JointSensor/1 -> Sign/1  "Velocity"
  Sign/1 -> Gain1/1
  JointSensor/3 -> Norm/1  "Reaction force (N)"
  Product/1 -> JointStictionActuator/5  "Reverse sliding stiction limit"
  Product2/1 -> JointStictionActuator/3  "Forward sliding stiction limit"
  Norm/1 -> Product3/2, Product2/1, Product/1
  Gain1/1 -> Product3/1
  Product3/1 -> JointStictionActuator/2, Kinetic Friction/1  "Kinetic friction"
  JointSensor/2 -> Sum2/1  "Computed torque"
  Sum2/1 -> JointStictionActuator/4, Static Friction/1  "Friction force"
  External Actuation/1 -> JointStictionActuator/1, Sum2/2
  connections:
  Mechanical Branching Bar/RConn2 -- JointStictionActuator/RConn1
  Mechanical Branching Bar/LConn1 -- To Joint/RConn1
  Mechanical Branching Bar/RConn1 -- JointSensor/LConn1

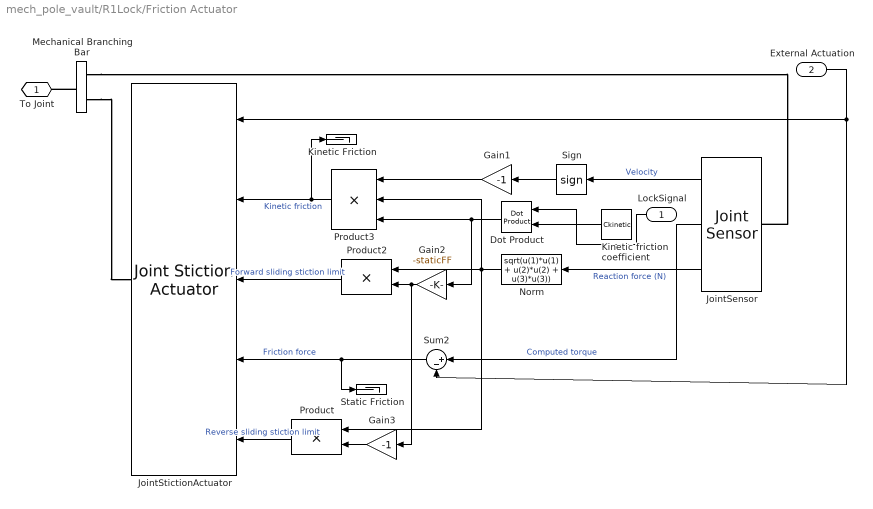
== system mech_pole_vault/R1Lock/Friction Actuator ==
  LockSignal : Inport  Orientation=left  OutDataType=sfix(16)  OutScaling=2^0
  External Actuation : Inport  Port=2  OutDataType=sfix(16)  OutScaling=2^0
  Dot Product : simulink/Math Operations/Dot Product  Orientation=left  InputSameDT=on  OutDataType=sfix(16)  OutScaling=2^-10  DoSatur=off
  Gain1 : Gain  Orientation=left  Gain=-1  ParameterDataType=sfix(16)  ParameterScaling=2^0  OutDataType=sfix(16)  OutScaling=2^0  SaturateOnIntegerOverflow=on  OutDataTypeStr=Inherit: Same as input  ParamDataTypeStr=Inherit: Same as input
  Gain2 : Gain  Orientation=left  Gain=-staticFF  ParameterDataType=sfix(16)  ParameterScaling=2^0  OutDataType=sfix(16)  OutScaling=2^0  SaturateOnIntegerOverflow=on  OutDataTypeStr=Inherit: Same as input  ParamDataTypeStr=Inherit: Same as input
  Gain3 : Gain  Orientation=left  Gain=-1  ParameterDataType=sfix(16)  ParameterScaling=2^0  OutDataType=sfix(16)  OutScaling=2^0  SaturateOnIntegerOverflow=on  OutDataTypeStr=Inherit: Same as input  ParamDataTypeStr=Inherit: Same as input
  JointSensor : mblibv1/Sensors &  Actuators/Joint Sensor  Orientation=left  DialogController=MECH.DynMechDlgSource  SystemSampleTime=-1  PhysicalDomain=Mechanical  PortType=blob  Muxed=off  Pose=off  Angle=off  AngleUnits=deg  ArcVelocity=on  ArcVelocityUnits=rad/s  ArcAcceleration=off  ArcAccelerationUnits=deg/s^2  CoordPosition=off  CoordPositionUnits=m  Velocity=on  VelocityUnits=m/s  Acceleration=off  AccelerationUnits=m/s^2  Quaternion=on  QuaternionDT=off  QuaternionDDT=off  QuaternionUnits=deg  OutputVector=[ 1 1 3 ]  ActiveIO=on  Width=5  DialogClass=MechanicalSensorBlock  Primitive=R1  Force=on  ForceUnits=N  Torque=on  TorqueUnits=N-m  ReferenceFrame=Absolute (INERTIAL)  ReactionSensedSide=Base  ReactionReferenceFrame=Absolute (World)  ReactionForce=on  ReactionForceUnits=N  ReactionMoment=off  ReactionMomentUnits=N-m
  JointStictionActuator : mblibv1/Sensors &  Actuators/Joint Stiction Actuator  Orientation=left  DialogController=MECH.DynMechDlgSource  SystemSampleTime=-1  PhysicalDomain=Mechanical  PortType=blob  ActuationStyle=Force  AngleUnits=deg  ArcVelocityUnits=deg/s  ArcAccelerationUnits=deg/s^2  CoordPositionUnits=m  VelocityUnits=m/s  AccelerationUnits=m/s^2  ForceUnits=N  TorqueUnits=N-m  ActiveIO=on  Width=5  DialogClass=EventActuatorBlock  Primitive=R1  FrictionalForceUnits=N  ExternalForceUnits=N  FrictionalTorqueUnits=N-m  ExternalTorqueUnits=N-m  LockingTolerance=1e-2
  Kinetic Friction : Terminator
  Kinetic friction  coefficient : Constant  Orientation=left  Value=Ckinetic  OutDataType=sfix(16)  OutScaling=2^0
  Mechanical Branching Bar : mblibv1/Utilities/Mechanical Branching Bar  DialogController=MECH.DynMechDlgSource  PhysicalDomain=mechanical  SubClassName=Unknown  LeftPortType=blob  RightPortType=blob  LConnTagsString=_newl0  RConnTagsString=SA0|SA1  DialogClass=MechanicalBranchingBarBlock  NumSAPorts=2
  Norm : Fcn  Orientation=left  Expr=sqrt(u(1)*u(1) + u(2)*u(2) + u(3)*u(3))
  Product : Product  Orientation=left  OutDataType=sfix(16)  OutScaling=2^0  SaturateOnIntegerOverflow=on  InputSameDT=on  OutDataTypeStr=Inherit: Same as first input
  Product2 : Product  Orientation=left  OutDataType=sfix(16)  OutScaling=2^0  SaturateOnIntegerOverflow=on  InputSameDT=on  OutDataTypeStr=Inherit: Same as first input
  Product3 : Product  Orientation=left  Inputs=3  OutDataType=sfix(16)  OutScaling=2^0  SaturateOnIntegerOverflow=on  InputSameDT=on  OutDataTypeStr=Inherit: Same as first input
  Sign : Signum  Orientation=left  ZeroCross=off
  Static Friction : Terminator
  Sum2 : Sum  Orientation=left  Inputs=|+-  OutDataType=sfix(16)  OutScaling=2^0  SaturateOnIntegerOverflow=on  InputSameDT=on  OutDataTypeStr=Inherit: Same as first input
  To Joint : PMIOPort  Port=1  Side=Right
  wires:
  External Actuation/1 -> Sum2/2, JointStictionActuator/1
  Sum2/1 -> Static Friction/1, JointStictionActuator/4  "Friction force"
  JointSensor/2 -> Sum2/1  "Computed torque"
  Product3/1 -> Kinetic Friction/1, JointStictionActuator/2  "Kinetic friction"
  Gain1/1 -> Product3/1
  Norm/1 -> Product/1, Product2/1, Product3/2
  Product2/1 -> JointStictionActuator/3  "Forward sliding stiction limit"
  Product/1 -> JointStictionActuator/5  "Reverse sliding stiction limit"
  JointSensor/3 -> Norm/1  "Reaction force (N)"
  Sign/1 -> Gain1/1
  JointSensor/1 -> Sign/1  "Velocity"
  Kinetic friction  coefficient/1 -> Dot Product/2
  Dot Product/1 -> Product3/3, Gain2/1
  LockSignal/1 -> Dot Product/1
  Gain2/1 -> Product2/2, Gain3/1
  Gain3/1 -> Product/2
  connections:
  Mechanical Branching Bar/RConn1 -- JointSensor/LConn1
  Mechanical Branching Bar/LConn1 -- To Joint/RConn1
  Mechanical Branching Bar/RConn2 -- JointStictionActuator/RConn1

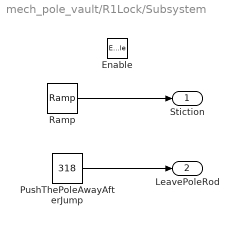
== system mech_pole_vault/R1Lock/Subsystem ==
  Enable : EnablePort
  PushThePoleAwayAfterJump : Constant  Value=318  OutDataType=sfix(16)  OutScaling=2^0
  Ramp : simulink/Sources/Ramp  SystemSampleTime=-1  slope=1  start=2.8  X0=0
  Stiction : Outport  OutDataType=sfix(16)  OutScaling=2^0
  LeavePoleRod : Outport  Port=2  OutDataType=sfix(16)  OutScaling=2^0  InitialOutput=0
  wires:
  Ramp/1 -> Stiction/1
  PushThePoleAwayAfterJump/1 -> LeavePoleRod/1
